simulink model "ziegler_nichols_odskocni_sim"  (R2020a)
settings: Solver=FixedStepAuto  StartTime=0.0  StopTime=sim_duration  FixedStep=time_step  RelTol=1e-3
undefined symbols (not defined in the file): C, E, L, R, t0, ue, x2e
settings Model: Creator=HP  LastModifiedBy=HP

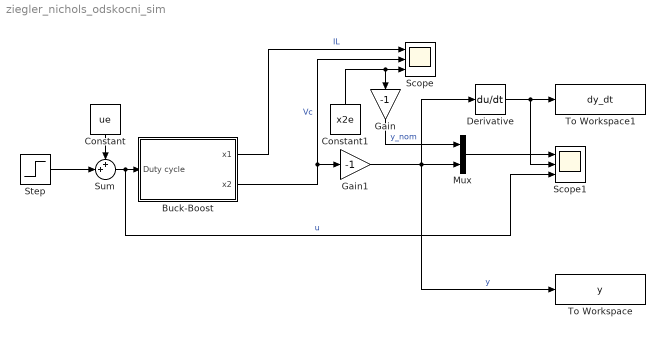
== system ziegler_nichols_odskocni_sim ==
  Buck-Boost : Subsystem
  Constant : Constant  Value=ue
  Constant1 : Constant  Value=x2e
  Derivative : Derivative
  Gain : Gain  Gain=-1
  Gain1 : Gain  Gain=-1
  Mux : Mux  Inputs=2
  Scope : Scope  NumInputPorts=3
  Scope1 : Scope  NumInputPorts=3
  Step : Step  Time=t0  After=0.1*ue  SampleTime=0
  Sum : Sum  Inputs=++|
  To Workspace : ToWorkspace  VariableName=y  SaveFormat=Timeseries  SampleTime=-1
  To Workspace1 : ToWorkspace  VariableName=dy_dt  SaveFormat=Timeseries  SampleTime=-1
  wires:
  Sum/1 -> Scope1/3, Buck-Boost/1(Duty cycle)  "u"
  Constant/1 -> Sum/1
  Step/1 -> Sum/2
  Constant1/1 -> Scope/3, Gain/1
  Buck-Boost/1(x1) -> Scope/1  "IL"
  Buck-Boost/2(x2) -> Gain1/1, Scope/2  "Vc"
  Gain/1 -> Mux/1  "y_nom"
  Gain1/1 -> To Workspace/1, Derivative/1, Mux/2  "y"
  Mux/1 -> Scope1/1
  Derivative/1 -> Scope1/2, To Workspace1/1

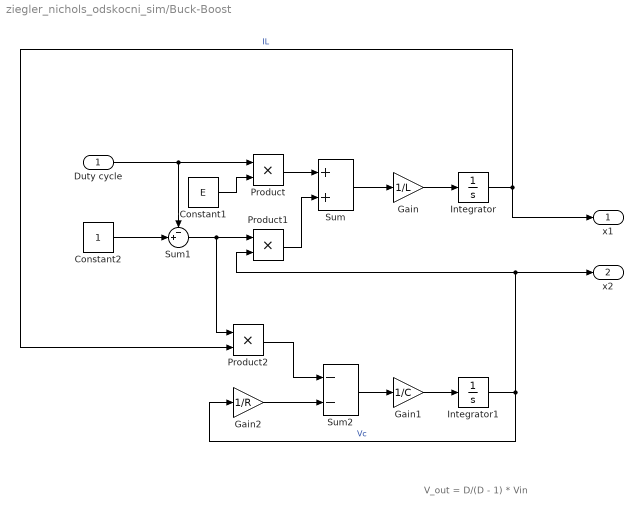
== system ziegler_nichols_odskocni_sim/Buck-Boost ==
  note: V_out = D/(D - 1) * Vin
  Duty cycle : Inport
  Constant1 : Constant  Value=E
  Constant2 : Constant
  Gain : Gain  Gain=1/L
  Gain1 : Gain  Gain=1/C
  Gain2 : Gain  Gain=1/R
  Integrator : Integrator
  Integrator1 : Integrator
  Product : Product
  Product1 : Product
  Product2 : Product
  Sum : Sum
  Sum1 : Sum  Inputs=-+|
  Sum2 : Sum  Inputs=--
  x1 : Outport
  x2 : Outport  Port=2
  wires:
  Product/1 -> Sum/1
  Product1/1 -> Sum/2
  Sum2/1 -> Gain1/1
  Constant1/1 -> Product/2
  Integrator1/1 -> Gain2/1, x2/1, Product1/2  "Vc"
  Gain1/1 -> Integrator1/1
  Constant2/1 -> Sum1/2
  Integrator/1 -> x1/1, Product2/2  "IL"
  Sum/1 -> Gain/1
  Gain2/1 -> Sum2/2
  Sum1/1 -> Product2/1, Product1/1
  Duty cycle/1 -> Sum1/1, Product/1
  Product2/1 -> Sum2/1
  Gain/1 -> Integrator/1
